simulink model "VendingMachineMealy"  (R2020b)
settings: Solver=VariableStepAuto  StartTime=0.0  StopTime=10.0  RelTol=1e-3
settings Model: Creator=DELL  LastModifiedBy=DELL

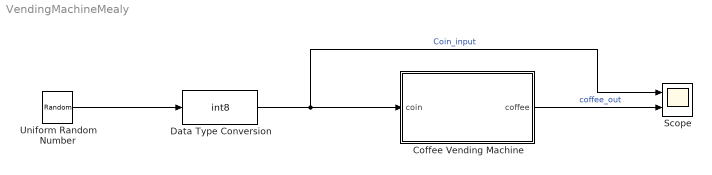
== system VendingMachineMealy ==
  Coffee Vending Machine : Stateflow chart  TreatAsAtomicUnit=on
  Data Type Conversion : DataTypeConversion  OutDataTypeStr=int8
  Scope : Scope  NumInputPorts=2
  Uniform Random Number : UniformRandomNumber  Minimum=0  Maximum=2  Seed=200  SampleTime=10
  wires:
  Uniform Random Number/1 -> Data Type Conversion/1
  Data Type Conversion/1 -> Scope/1, Coffee Vending Machine/1(coin)  "Coin_input"
  Coffee Vending Machine/1(coffee) -> Scope/2  "coffee_out"

== stateflow chart VendingMachineMealy/Coffee Vending Machine ==
  state Got_5_rs
  state Got_0_rs
  state Got_10_rs
  (default) -> Got_0_rs
  Got_0_rs -> Got_5_rs [order 1] : [coin==1]{coffee=0;}
  Got_5_rs -> Got_0_rs [order 1] : [coin==2]{coffee=1;}
  Got_10_rs -> Got_0_rs [order 1] : [coin==1]{coffee=1;}
  Got_0_rs -> Got_10_rs [order 2] : [coin==2]{coffee=0;}
  Got_10_rs -> Got_5_rs [order 2] : [coin==2]{coffee=1;}
  Got_5_rs -> Got_10_rs [order 2] : [coin==1]{coffee=0;}
  data: coin input; coffee output
